simulink model "Raspi_2layers"  (R2021b)
settings: Solver=FixedStepDiscrete  StartTime=0.0  StopTime=inf  FixedStep=1e-2  RelTol=1e-3  EnableMultiTasking=on
libraries: raspberrypiNetworklib x4
settings Model: Creator=Blade  LastModifiedBy=Blade
settings SolverCC: PositivePriorityOrder=on
settings OptimizationCC: EnhancedBackFolding=on  PassReuseOutputArgsAs=Individual arguments  ZeroExternalMemoryAtStartup=off  ZeroInternalMemoryAtStartup=off  MaxStackSize=64  OptimizeBlockOrder=speed  DifferentSizesBufferReuse=on  OptimizationCustomize=off  EfficientTunableParamExpr=on
settings DebuggingCC: ParameterTunabilityLossMsg=error
settings HardwareCC: ProdBitPerPointer=32  ProdBitPerSizeT=32  ProdBitPerPtrDiffT=32  ProdLargestAtomicInteger=Long  ProdLargestAtomicFloat=Double  ProdWordSize=32  ProdLongLongMode=on  ProdHWDeviceType=ARM Compatible->ARM Cortex
settings RTWCC: Description=Embedded Coder  SystemTargetFile=ert.tlc  HardwareBoard=Raspberry Pi  TLCOptions="-aInlineSetEventsForThisBaseRateFcn=TLC_FALSE -aSuppressMultiTaskScheduler=TLC_FALSE  -aRateBasedStepFcn=0"  TemplateMakefile=ert_default_tmf  Toolchain=GNU GCC Embedded Linux  BuildConfiguration=Faster Runs
settings CodeAppCC: ForceParamTrailComments=on  IgnoreCustomStorageClasses=off  OperatorAnnotations=on  SimulinkDataObjDesc=on  SFDataObjDesc=on  InsertBlockDesc=on
settings ERTTargetCC: SupportContinuousTime=on  SupportVariableSizeSignals=on  ExtModeTransport=2  ExtModeStaticAlloc=on  ExtModeMexFile=ext_xcp  ExtModeIntrfLevel=Level2 - Open

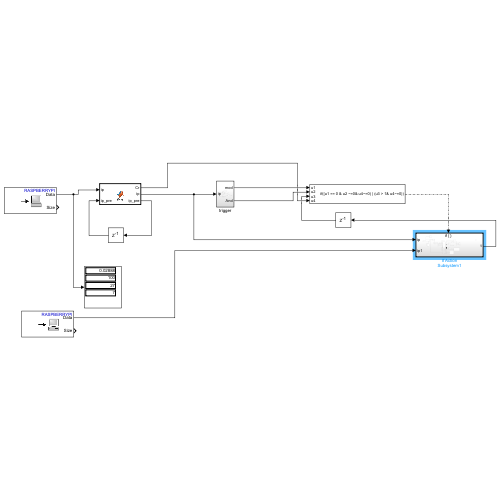
[thumbnail: Simulink's stored preview of the top-level diagram]
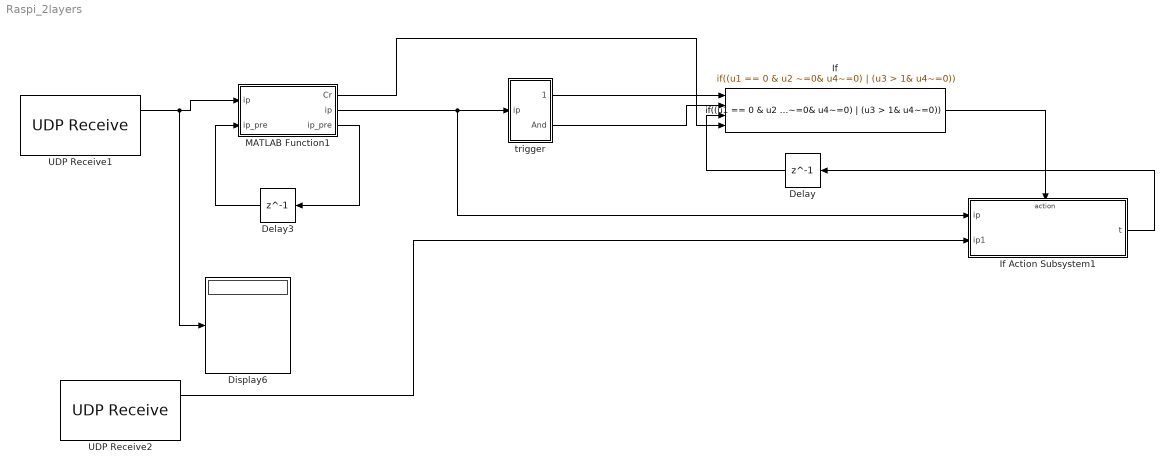
== system Raspi_2layers ==
  Delay : Delay  DelayLength=1  InitialCondition=0
  Delay3 : Delay  DelayLength=1  InitialCondition=0
  Display6 : Display
  If : If  NumInputs=4  IfExpression=(u1 == 0 & u2 ~=0& u4~=0) | (u3 > 1& u4~=0)  ShowElse=off
  If Action Subsystem1 : Subsystem  TreatAsAtomicUnit=on
  MATLAB Function1 : MATLAB Function  TreatAsAtomicUnit=on
  UDP Receive1 : raspberrypiNetworklib/UDP Receive  localURL='0.0.0.0'  localPort=1000  remoteURL='0.0.0.0'  remotePort=-1  recvBufferSize=8192  signalDatatype=double  dims=4  isVarSize=off  showBlockingTime=off  blockingTime=0  sampletime=-1  blockPlatform=Raspberry Pi
      settings: SourceProductBaseCode=RASPPI
  UDP Receive2 : raspberrypiNetworklib/UDP Receive  localURL='0.0.0.0'  localPort=1100  remoteURL='0.0.0.0'  remotePort=-1  recvBufferSize=8192  signalDatatype=double  dims=4  isVarSize=off  showBlockingTime=off  blockingTime=0  sampletime=-1  blockPlatform=Raspberry Pi
      settings: SourceProductBaseCode=RASPPI
  trigger : Subsystem
  wires:
  MATLAB Function1/1(Cr) -> If/4
  trigger/1(mod) -> If/1
  Delay3/1 -> MATLAB Function1/2("ip_pre ")
  UDP Receive1/1 -> Display6/1, MATLAB Function1/1("ip ")
  trigger/2(And) -> If/2
  MATLAB Function1/2(ip) -> If Action Subsystem1/1(ip), trigger/1(ip)
  Delay/1 -> If/3
  MATLAB Function1/3(ip_pre) -> Delay3/1
  If Action Subsystem1/1(t) -> Delay/1
  UDP Receive2/1 -> If Action Subsystem1/2(ip1)
  If/1 -> If Action Subsystem1/Action

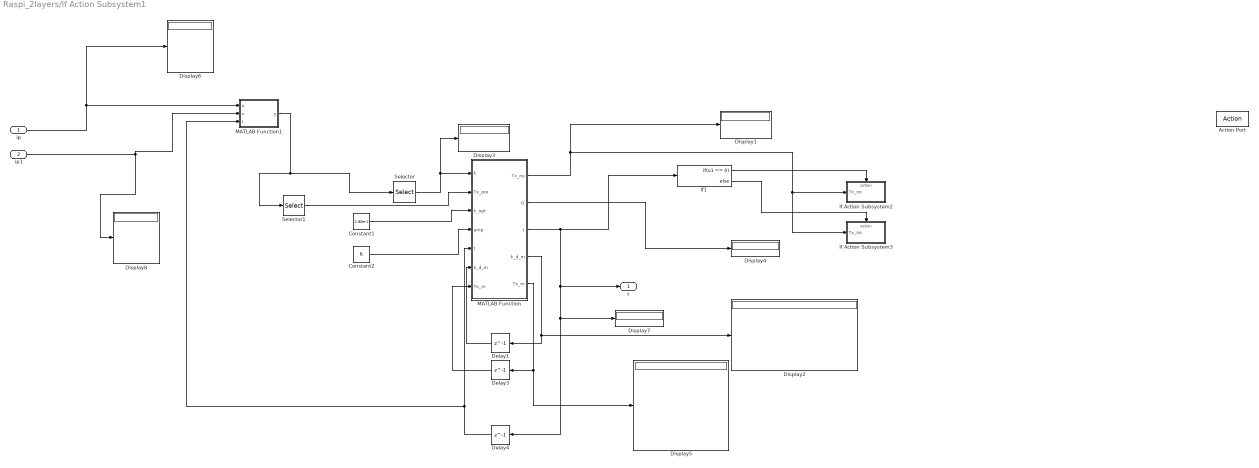
== system Raspi_2layers/If Action Subsystem1 ==
  ip : Inport
  ip1 : Inport  Port=2
  Action Port : ActionPort  ActionPortLabel=if((u1 == 0 & u2 ~=0& u4~=0) | (u3 > 1& u4~=0))
  Constant1 : Constant  Value=2.88e-2
  Constant2 : Constant  Value=6
  Delay1 : Delay  DelayLength=1  InitialCondition=zeros(2,3)
  Delay3 : Delay  DelayLength=1  InitialCondition=zeros(8,2)
  Delay4 : Delay  DelayLength=1  InitialCondition=0
  Display{1..8} (8 alike) : Display
  If Action Subsystem2 : Subsystem  TreatAsAtomicUnit=on
  If Action Subsystem3 : Subsystem  TreatAsAtomicUnit=on
  If1 : If  IfExpression=u1 == 0
  MATLAB Function : MATLAB Function  TreatAsAtomicUnit=on
  MATLAB Function1 : MATLAB Function  TreatAsAtomicUnit=on
  Selector : Selector  InputPortWidth=4  IndexOptions=Index vector (dialog)  Indices=1  OutputSizes=1
  Selector1 : Selector  InputPortWidth=4  IndexOptions=Index vector (dialog)  Indices=[3;4]  OutputSizes=1
  t : Outport
  wires:
  MATLAB Function/5(Tx_m) -> Display5/1, Delay3/1
  MATLAB Function/2(G) -> Display4/1
  MATLAB Function/4(k_d_m) -> Delay1/1, Display2/1
  Delay1/1 -> MATLAB Function/6("k_d_m ")
  Selector/1 -> Display3/1, MATLAB Function/1(k)
  MATLAB Function/3(t) -> If1/1, Display7/1, Delay4/1, t/1
  Delay4/1 -> MATLAB Function1/3(t), MATLAB Function/5("t ")
  MATLAB Function/1(Tx_no) -> If Action Subsystem3/1(Tx_no), If Action Subsystem2/1(Tx_no), Display1/1
  Constant2/1 -> MATLAB Function/4(amp)
  Selector1/1 -> MATLAB Function/2(Tx_pre)
  Delay3/1 -> MATLAB Function/7("Tx_m ")
  MATLAB Function1/1(y) -> Selector1/1, Selector/1
  Constant1/1 -> MATLAB Function/3(k_opt)
  ip/1 -> MATLAB Function1/1(u), Display6/1
  If1/1 -> If Action Subsystem2/Action
  If1/2 -> If Action Subsystem3/Action
  ip1/1 -> Display8/1, MATLAB Function1/2(v)

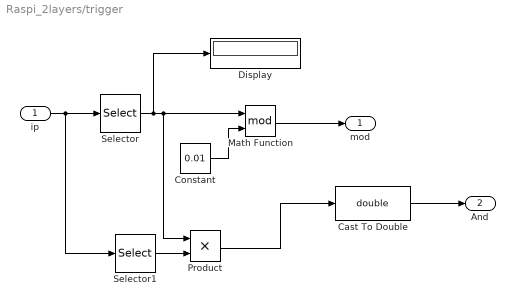
== system Raspi_2layers/trigger ==
  ip : Inport
  Cast To Double : DataTypeConversion  OutDataTypeStr=double
  Constant : Constant  Value=0.01
  Display : Display
  Math Function : Math  Operator=mod  SaturateOnIntegerOverflow=on
  Product : Product
  Selector : Selector  InputPortWidth=4  IndexOptions=Index vector (dialog)  Indices=2  OutputSizes=1
  Selector1 : Selector  InputPortWidth=4  IndexOptions=Index vector (dialog)  Indices=1  OutputSizes=1
  mod : Outport
  And : Outport  Port=2
  wires:
  Constant/1 -> Math Function/2
  Selector/1 -> Display/1, Product/1, Math Function/1
  ip/1 -> Selector1/1, Selector/1
  Math Function/1 -> mod/1
  Product/1 -> Cast To Double/1
  Selector1/1 -> Product/2
  Cast To Double/1 -> And/1

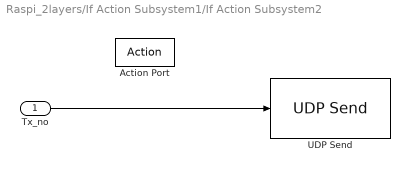
== system Raspi_2layers/If Action Subsystem1/If Action Subsystem2 ==
  Tx_no : Inport
  Action Port : ActionPort  ActionPortLabel=if(u1 == 0)
  UDP Send : raspberrypiNetworklib/UDP Send  remoteURL='172.20.10.2'  remotePort=2000  localURL='0.0.0.0'  localPortSource=Automatically determine  localPort=-1  sampletime=-1  blockPlatform=Raspberry Pi  separateLengthPort=0
      settings: SourceProductBaseCode=RASPPI
  wires:
  Tx_no/1 -> UDP Send/1

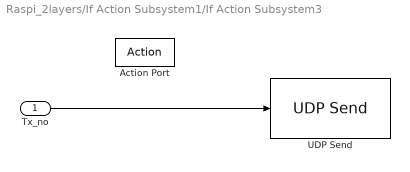
== system Raspi_2layers/If Action Subsystem1/If Action Subsystem3 ==
  Tx_no : Inport
  Action Port : ActionPort  ActionPortLabel=else
  UDP Send : raspberrypiNetworklib/UDP Send  remoteURL='172.20.10.2'  remotePort=2100  localURL='0.0.0.0'  localPortSource=Automatically determine  localPort=-1  sampletime=-1  blockPlatform=Raspberry Pi  separateLengthPort=0
      settings: SourceProductBaseCode=RASPPI
  wires:
  Tx_no/1 -> UDP Send/1

== matlab function Raspi_2layers/MATLAB Function1 ==
  data: Cr output; ip output; ip input; ip_pre input; ip_pre output
function [Cr,ip, ip_pre] = fcn(ip, ip_pre)

ip2 = ip(2);

if ip2 == ip_pre
    Cr = 0;
else
    ip_pre = ip2;
    Cr = 1;

end

== matlab function Raspi_2layers/If Action Subsystem1/MATLAB Function1 ==
  data: u input; y output; v input; t input
function y = IpSelector(u,v,t)
if t<=2
    y = u;
else
    y = v;
end

== matlab function Raspi_2layers/If Action Subsystem1/MATLAB Function ==
  data: k input; Tx_pre input; Tx_no output; G output; t output; k_opt input; amp input; t input; k_d_m output; k_d_m input; Tx_m input; Tx_m output
function [Tx_no,G,t,k_d_m,Tx_m] = Controller(k,Tx_pre,k_opt,amp,t,k_d_m,Tx_m)

k_diff = abs(k_opt-k)/k_opt;
Tx_pre = Tx_pre';

if t == 0
   

    t = t+1;
    k_d_m(1,:)  = [k_diff,Tx_pre];
    k_d_m(2,:)  = [k_diff,Tx_pre];

    
else

    if k_diff < k_d_m(2,1)

       k_d_m(2,:)  = [k_diff,Tx_pre];

    end

end

G = round(amp*k_d_m(1,1));  
Tx_fix = k_d_m(1,2:3)';

if G >1
    G =1;
    disp("Gain exceed!!!")
end

if t < 10
    
    if t < 9

        if G ==0
            Tx_no = [0;0];
        else

            dir_att = [-1,-1; -1,0; 0,-1; 1,1; 1,0; 0,1; 1,-1; -1,1];
            
            
            Tx_no =G*dir_att(t,:)'+Tx_fix;
        
            Tx_m (t,:) = Tx_no;
        end

    else

         Tx_no = [0;0]; % off

    end

    t =t+1;

else
    
    
    Tx_no = k_d_m(2,2:3)';

    t =0;
   
 
end
